simulink model "Dfig"  (R2017b)
settings: Solver=ode45  StartTime=0.0  StopTime=20  RelTol=1e-3  EnableMultiTasking=on
undefined symbols (not defined in the file): D, DiscIntNeverNeededParam, f, Fs, fsw, J, ki_id, ki_n, kp_id, kp_n, Lm, Lr, Ls, Lsi, p, Ps, Rr, Rs, sigma, Tem, Ts, Vbus, Vs
libraries: powerlib x8, powerlib_meascontrol x1
settings Model: Creator=admin  LastModifiedBy=admin
settings DataIOCC: LimitDataPoints=on  SaveFormat=Array
settings OptimizationCC: LifeSpan=inf
settings DebuggingCC: UnderspecifiedInitializationDetection=Classic  MergeDetectMultiDrivingBlocksExec=none  SolverPrmCheckMsg=warning  StateNameClashWarn=warning  SFUnexpectedBacktrackingDiag=warning  SFNoUnconditionalDefaultTransitionDiag=warning  SFExecutionAtInitializationDiag=none
settings HardwareCC: ProdBitPerPointer=32  ProdBitPerSizeT=32  ProdBitPerPtrDiffT=32  ProdLargestAtomicFloat=None  ProdIntDivRoundTo=Undefined  ProdEndianess=Unspecified  ProdWordSize=32  ProdHWDeviceType=32-bit Generic
settings ModelReferenceCC: PropagateSignalLabelsOutOfModel=off
settings CodeAppCC: StateflowObjectComments=on
settings GRTTargetCC: TargetLangStandard=C89/C90 (ANSI)  GeneratePreprocessorConditionals=Disable all
settings ConfigComp: CovMetricSettings=dw  CovHtmlReporting=on  CovSaveCumulativeToWorkspaceVar=on  CovSaveSingleToWorkspaceVar=on  CovExternalEMLEnable=off
settings SimscapeCC: SimscapeNormalizeSystem=off

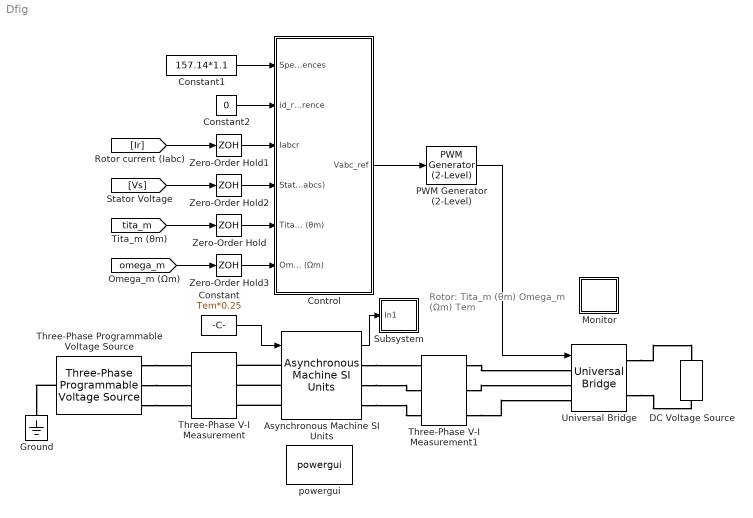
== system Dfig ==
  note: Rotor:
      | Tita_m (θm)
      | Omega_m (Ωm)
      | Tem
  Asynchronous Machine SI Units : powerlib/Machines/Asynchronous Machine SI Units  RotorType=Wound  PresetModel=No  MechanicalLoad=Torque Tm  ShowDetailedParameters=on  ReferenceFrame=Rotor  Units=SI  MeasurementBus=off  NominalParameters=[ Ps Vs f ]  Stator=[ Rs , Lsi]  Rotor=[ Rr , Lsi]  Cage1=[ 0.022 0.226/377]  Cage2=[ 0.022 0.226/377]  Lm=Lm  Mechanical=[ J D 2 ]  PolePairs=2  InitialConditions=[1 0 0 0 0 0 0 0]  SimulateSaturation=off  Saturation=[14.03593122, 27.81365428, 53.79336849, 72.68890987, 97.98006896, 148.6815601, 215.7428561, 302.9841135, 420.4778367 ; 230, 322, 414, 460, 506, 552, 598, 644, 690]  LoadFlowParameters=1492000  TsPowergui=0  TsBlock=-1  IterativeModel=Trapezoidal non iterative  IterativeDiscreteModel=Trapezoidal non iterative  Pmec=0
  Constant : Constant  Value=Tem*0.25
  Constant1 : Constant  Value=157.14*1.1
  Constant2 : Constant  Value=0
  Control : Subsystem
  DC Voltage Source : powerlib/Electrical Sources/DC Voltage Source  Amplitude=Vbus  Measurements=None
  Ground : powerlib/Elements/Ground  LConnTagsString=a
  Monitor : Subsystem
  PWM Generator (2-Level) : powerlib_meascontrol/Pulse & Signal Generators/PWM Generator (2-Level)  ModulatorType=Three-phase bridge (6 pulses)  ModulatorMode=Unsynchronized  Fc=fsw  Pc=90  nF=27  MinMax="[ -1  1 ]"  SamplingTechnique=Natural  ModulatingSignals=off  m=0.8  Freq=60  Phase=0  Ts=0  ShowCarrierOutport=off
      settings: SourceProductName=Simscape Power Systems
  Subsystem : Subsystem
  Three-Phase Programmable Voltage Source : powerlib/Electrical Sources/Three-Phase Programmable Voltage Source  PositiveSequence="[Vs  0 f]"  VariationEntity=None  VariationType=Table of time-amplitude pairs  VariationTypeAlt=Step  VariationStep=0.5  VariationRate=10  VariationMagnitude=0.3  VariationFrequency=2  VariationTiming=[1 2]  VariationPhaseA=off  Amplitudes=[1 0.8 1.2 1.0]  TimeValues=[0 0.1 0.15 0.2]  HarmonicGeneration=off  HarmonicA=[3 0.2 -25 0]  HarmonicB=[2 0.15 35 2]  Timing="[0.05  3]"  BusType=swing  Pref=0  Qref=0  Qmin=-inf  Qmax=inf
  Three-Phase V-I Measurement : powerlib/Measurements/Three-Phase V-I Measurement  VoltageMeasurement=phase-to-ground  SetLabelV=on  LabelV=Vs  Vpu=off  VpuLL=off  CurrentMeasurement=yes  SetLabelI=on  LabelI=Is  Ipu=off  Pbase=100e6  Vbase=500e3  OutputType=Complex  PhasorSimulation=off  PSBequivalent=0
  Three-Phase V-I Measurement1 : powerlib/Measurements/Three-Phase V-I Measurement  VoltageMeasurement=phase-to-phase  SetLabelV=on  LabelV=Vr  Vpu=off  VpuLL=off  CurrentMeasurement=yes  SetLabelI=on  LabelI=Ir  Ipu=off  Pbase=100e6  Vbase=500e3  OutputType=Complex  PhasorSimulation=off  PSBequivalent=0
  Universal Bridge : powerlib/Power Electronics/Universal Bridge  Arms=3  SnubberResistance=1e5  SnubberCapacitance=inf  Device=Ideal Switches  Ron=1e-3  Lon=0  ForwardVoltages="[  0  0  ]"  ForwardVoltage=0  GTOparameters=[ 10e-6 , 20e-6 ]  IGBTparameters=[ 1e-6 , 2e-6 ]  Measurements=None  Measurements_2=None  converterType=Rectifier
  Zero-Order Hold{,1..3} (4 alike) : ZeroOrderHold  SampleTime=1/fsw
  powergui : powerlib/powergui  Priority=1  SimulationMode=Discrete  SampleTime=Ts  frequency=60  Iterations=50  frequencyindice=50  Pbase=100e6  ErrMax=1e-4  UnitsV=kV  UnitsW=MW  buscounter=0  FunctionMessages=off  echomessages=off  EnableUseOfTLC=off  CurrentSourceSwitches=off  DisableSnubberDevices=off  DisableRonSwitches=off  DisableVfSwitches=off  DisplayEquations=off  SolverType=Tustin  Interpol=off  ExternalGateDelay=off  methode=off  Ts=0  x0status=blocks  SPID=off  SwTol=0  HookPort=off  RestoreLinks=warning  ResistiveCurrentMeasurement=off  Frange=[0:2:500]  Ylog=off  Xlog=on  ShowGrid=off  save=off  variable=ZData  structure=0  ZoomFFT=off  StartTime=0.0  cycles=1  DisplayStyle=1  fundamental=60  FreqAxis=off  MaxFrequency=1000  frequencyindicesteady=1  RmsSteady=1  display=off
  wires:
  Constant/1 -> Asynchronous Machine SI Units/1
  PWM Generator (2-Level)/1 -> Universal Bridge/1
  Control/1(Vabc_ref) -> PWM Generator (2-Level)/1
  Constant1/1 -> Control/1(Speed reference Omega_m (Ωm) references)
  Constant2/1 -> Control/2(id_reference)
  [Vs] -> Zero-Order Hold2/1
  [Ir] -> Zero-Order Hold1/1
  Asynchronous Machine SI Units/1 -> Subsystem/1(In1)
  [tita_m] -> Zero-Order Hold/1
  [omega_m] -> Zero-Order Hold3/1
  Zero-Order Hold1/1 -> Control/3(Iabcr)
  Zero-Order Hold2/1 -> Control/4(Stator Voltage (Vabcs))
  Zero-Order Hold/1 -> Control/5(Tita_m (θm))
  Zero-Order Hold3/1 -> Control/6(Omega_m (Ωm))
  connections:
  Three-Phase Programmable Voltage Source/LConn1 -- Ground/LConn1
  Three-Phase Programmable Voltage Source/RConn1 -- Three-Phase V-I Measurement/LConn1
  Three-Phase Programmable Voltage Source/RConn2 -- Three-Phase V-I Measurement/LConn2
  Three-Phase Programmable Voltage Source/RConn3 -- Three-Phase V-I Measurement/LConn3
  Asynchronous Machine SI Units/LConn1 -- Three-Phase V-I Measurement/RConn1
  Asynchronous Machine SI Units/LConn2 -- Three-Phase V-I Measurement/RConn2
  Asynchronous Machine SI Units/LConn3 -- Three-Phase V-I Measurement/RConn3
  Universal Bridge/RConn2 -- DC Voltage Source/LConn1
  Universal Bridge/RConn1 -- DC Voltage Source/RConn1
  Asynchronous Machine SI Units/RConn1 -- Three-Phase V-I Measurement1/RConn1
  Asynchronous Machine SI Units/RConn2 -- Three-Phase V-I Measurement1/RConn2
  Asynchronous Machine SI Units/RConn3 -- Three-Phase V-I Measurement1/RConn3
  Three-Phase V-I Measurement1/LConn1 -- Universal Bridge/LConn1
  Three-Phase V-I Measurement1/LConn2 -- Universal Bridge/LConn2
  Three-Phase V-I Measurement1/LConn3 -- Universal Bridge/LConn3

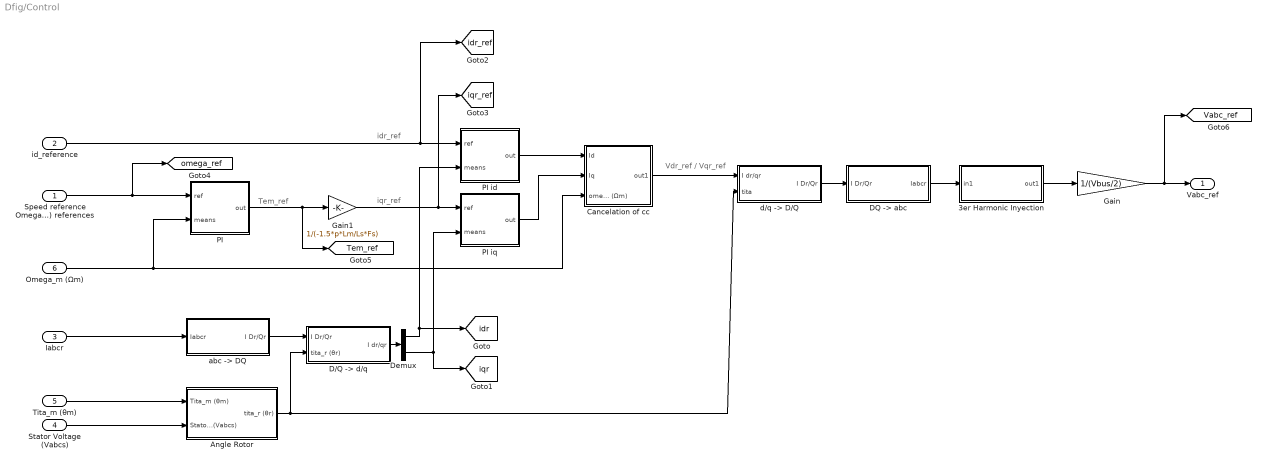
== system Dfig/Control ==
  note: Vdr_ref / Vqr_ref
  note: iqr_ref
  note: Tem_ref
  note: idr_ref
  Speed reference Omega_m (Ωm) references : Inport
  id_reference : Inport  Port=2
  Iabcr : Inport  Port=3
  Stator Voltage (Vabcs) : Inport  Port=4
  Tita_m (θm) : Inport  Port=5
  Omega_m (Ωm) : Inport  Port=6
  " Angle Rotor" : Subsystem
  3er Harmonic Inyection : Subsystem
  Cancelation of cc : Subsystem
  "D/Q -> d/q" : Subsystem
  "DQ -> abc" : Subsystem
  Demux : Demux  Outputs=2
  Gain : Gain  Gain=1/(Vbus/2)
  Gain1 : Gain  Gain=1/(-1.5*p*Lm/Ls*Fs)
  PI : Subsystem
  PI id : Subsystem
  PI iq : Subsystem
  "abc -> DQ " : Subsystem
  "d/q -> D/Q " : Subsystem
  Vabc_ref : Outport
  tag scope: Tem_ref=global, Vabc_ref=global, idr=global, idr_ref=global, iqr=global, iqr_ref=global, omega_ref=global
  wires:
  Gain/1 -> [Vabc_ref], Vabc_ref/1
  "DQ -> abc"/1(Iabcr) -> 3er Harmonic Inyection/1(in1)
  "d/q -> D/Q "/1(I Dr/Qr) -> "DQ -> abc"/1(I Dr/Qr)
  Iabcr/1 -> "abc -> DQ "/1(Iabcr)
  "abc -> DQ "/1(I Dr/Qr) -> "D/Q -> d/q"/1(I Dr/Qr)
  3er Harmonic Inyection/1(out1) -> Gain/1
  Tita_m (θm)/1 -> " Angle Rotor"/1(Tita_m (θm))
  Stator Voltage (Vabcs)/1 -> " Angle Rotor"/2(Stator Voltage (Vabcs))
  " Angle Rotor"/1(tita_r (θr)) -> "D/Q -> d/q"/2(tita_r (θr)), "d/q -> D/Q "/2(tita)
  PI id/1(out) -> Cancelation of cc/1(Id)
  PI iq/1(out) -> Cancelation of cc/2(Iq)
  Omega_m (Ωm)/1 -> PI/2(means), Cancelation of cc/3(omega_m (Ωm))
  "D/Q -> d/q"/1(I dr/qr) -> Demux/1
  Demux/2 -> [iqr], PI iq/2(means)
  Demux/1 -> [idr], PI id/2(means)
  Speed reference Omega_m (Ωm) references/1 -> PI/1(ref), [omega_ref]
  PI/1(out) -> [Tem_ref], Gain1/1
  Gain1/1 -> [iqr_ref], PI iq/1(ref)
  id_reference/1 -> [idr_ref], PI id/1(ref)
  Cancelation of cc/1(out1) -> "d/q -> D/Q "/1(I dr/qr)

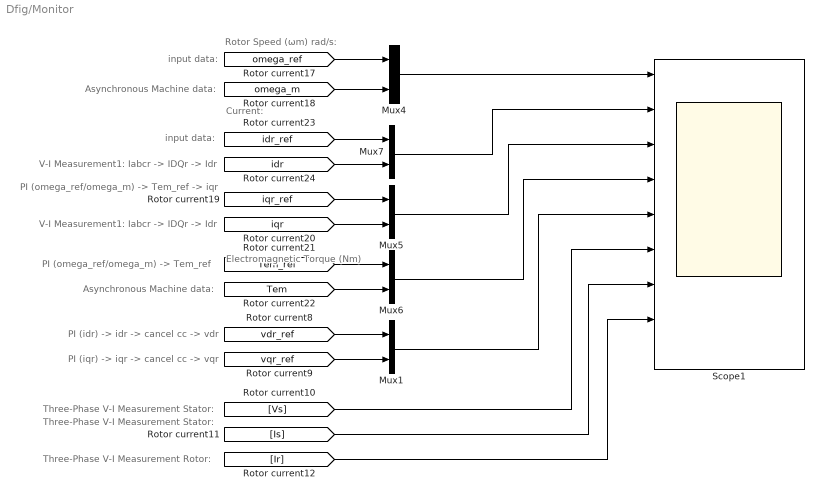
== system Dfig/Monitor ==
  note: Electromagnetic Torque (Nm)
  note: Three-Phase V-I Measurement Stator:
  note: PI (idr) -> idr -> cancel cc -> vdr
  note: PI (omega_ref/omega_m) -> Tem_ref -> iqr
  note: V-I Measurement1: Iabcr -> IDQr -> Idr
  note: input data:
  note: Current:
  note: Rotor Speed (ωm) rad/s:
  note: Asynchronous Machine data:
  note: input data:
  note: V-I Measurement1: Iabcr -> IDQr -> Idr
  note: PI (omega_ref/omega_m) -> Tem_ref
  note: Asynchronous Machine data:
  note: PI (iqr) -> iqr -> cancel cc -> vqr
  note: Three-Phase V-I Measurement Stator:
  note: Three-Phase V-I Measurement Rotor:
  Mux{1,4..7} (5 alike) : Mux  Inputs=2
  Scope1 : Scope  NumInputPorts=9
  wires:
  [omega_m] -> Mux4/2
  [omega_ref] -> Mux4/1
  [iqr_ref] -> Mux5/1
  [iqr] -> Mux5/2
  [Tem] -> Mux6/2
  [Tem_ref] -> Mux6/1
  [idr] -> Mux7/2
  [idr_ref] -> Mux7/1
  Mux4/1 -> Scope1/1
  [vdr_ref] -> Mux1/1
  [vqr_ref] -> Mux1/2
  Mux7/1 -> Scope1/2
  Mux5/1 -> Scope1/3
  Mux6/1 -> Scope1/4
  Mux1/1 -> Scope1/5
  [Vs] -> Scope1/6
  [Is] -> Scope1/7
  [Ir] -> Scope1/8

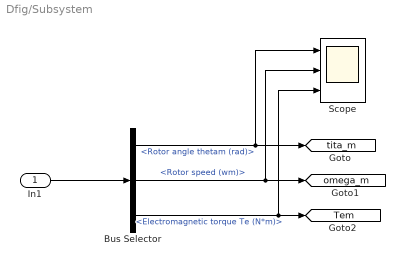
== system Dfig/Subsystem ==
  In1 : Inport
  Bus Selector : BusSelector  OutputSignals=Mechanical.Rotor angle thetam (rad),Mechanical.Rotor speed (wm),Mechanical.Electromagnetic torque Te (N*m)
  Scope : Scope  NumInputPorts=3
  tag scope: Tem=global, omega_m=global, tita_m=global
  wires:
  Bus Selector/2 -> Scope/2, [omega_m]  "<Rotor speed (wm)>"
  In1/1 -> Bus Selector/1
  Bus Selector/1 -> Scope/1, [tita_m]  "<Rotor angle thetam (rad)>"
  Bus Selector/3 -> Scope/3, [Tem]  "<Electromagnetic torque Te (N*m)>"

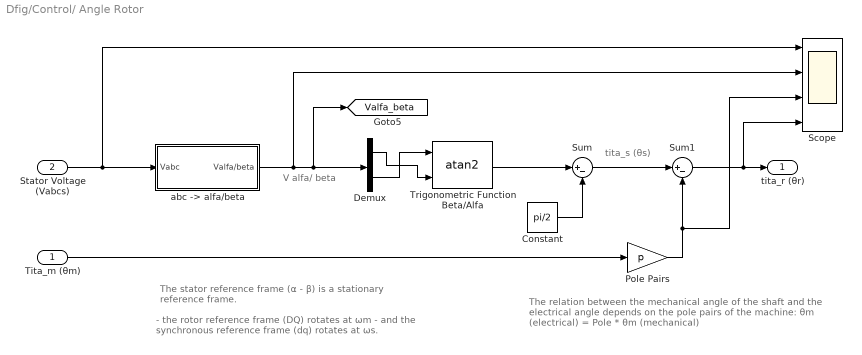
== system Dfig/Control/ Angle Rotor ==
  note: - the rotor reference frame (DQ) rotates at ωm
      | - and the synchronous reference frame (dq) rotates at ωs.
  note: The stator reference frame (α - β) is a stationary
      | reference frame.
  note: The relation between the mechanical angle of the shaft  and the
      | electrical angle depends on the pole pairs of the machine:
      |
      | θm (electrical) = Pole * θm (mechanical)
  note: tita_s (θs)
  note: V alfa/ beta
  Tita_m (θm) : Inport
  Stator Voltage (Vabcs) : Inport  Port=2
  Constant : Constant  Value=pi/2
  Demux : Demux  Outputs=2
  Pole Pairs : Gain  Gain=p
  Scope : Scope  NumInputPorts=4
  Sum : Sum  Inputs=|+-
  Sum1 : Sum  Inputs=|+-
  Trigonometric Function Beta/Alfa : Trigonometry  Operator=atan2
  "abc -> alfa/beta " : Subsystem
  tita_r (θr) : Outport
  tag scope: Valfa_beta=global
  wires:
  Stator Voltage (Vabcs)/1 -> Scope/1, "abc -> alfa/beta "/1(Vabc)
  Demux/2 -> Trigonometric Function Beta/Alfa/1
  Demux/1 -> Trigonometric Function Beta/Alfa/2
  "abc -> alfa/beta "/1("Valfa/beta ") -> Scope/2, [Valfa_beta], Demux/1
  Trigonometric Function Beta/Alfa/1 -> Sum/1
  Constant/1 -> Sum/2
  Tita_m (θm)/1 -> Pole Pairs/1
  Sum/1 -> Sum1/1
  Sum1/1 -> Scope/4, tita_r (θr)/1
  Pole Pairs/1 -> Sum1/2, Scope/3

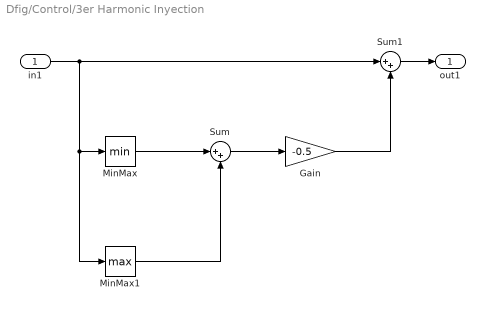
== system Dfig/Control/3er Harmonic Inyection ==
  in1 : Inport
  Gain : Gain  Gain=-0.5
  MinMax : MinMax
  MinMax1 : MinMax  Function=max
  Sum : Sum  Inputs=|++
  Sum1 : Sum  Inputs=|++
  out1 : Outport
  wires:
  in1/1 -> Sum1/1, MinMax1/1, MinMax/1
  MinMax/1 -> Sum/1
  MinMax1/1 -> Sum/2
  Sum1/1 -> out1/1
  Sum/1 -> Gain/1
  Gain/1 -> Sum1/2

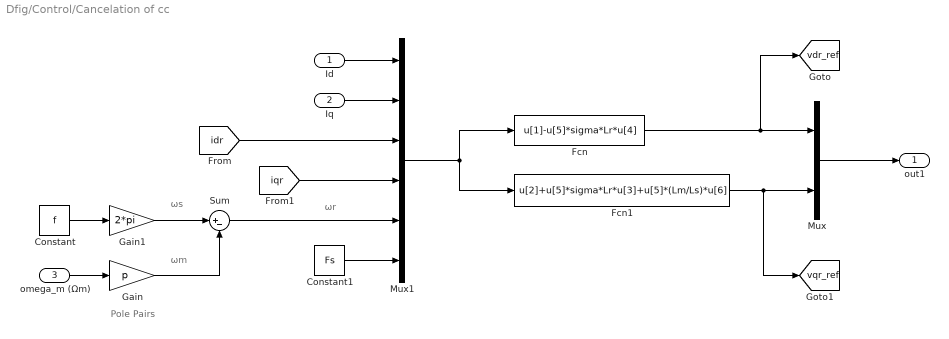
== system Dfig/Control/Cancelation of cc ==
  note: Pole Pairs
  note: ωr
  note: ωm
  note: ωs
  Id : Inport
  Iq : Inport  Port=2
  omega_m (Ωm) : Inport  Port=3
  Constant : Constant  Value=f
  Constant1 : Constant  Value=Fs
  Fcn : Fcn  Expr=u[1]-u[5]*sigma*Lr*u[4]
  Fcn1 : Fcn  Expr=u[2]+u[5]*sigma*Lr*u[3]+u[5]*(Lm/Ls)*u[6]
  Gain : Gain  Gain=p
  Gain1 : Gain  Gain=2*pi
  Mux : Mux  Inputs=2
  Mux1 : Mux  Inputs=6
  Sum : Sum  Inputs=|+-
  out1 : Outport
  tag scope: vdr_ref=global, vqr_ref=global
  wires:
  Mux/1 -> out1/1
  Fcn/1 -> [vdr_ref], Mux/1
  Fcn1/1 -> [vqr_ref], Mux/2
  Id/1 -> Mux1/1
  Iq/1 -> Mux1/2
  Mux1/1 -> Fcn1/1, Fcn/1
  [idr] -> Mux1/3
  [iqr] -> Mux1/4
  Constant1/1 -> Mux1/6
  omega_m (Ωm)/1 -> Gain/1
  Gain/1 -> Sum/2
  Constant/1 -> Gain1/1
  Gain1/1 -> Sum/1
  Sum/1 -> Mux1/5

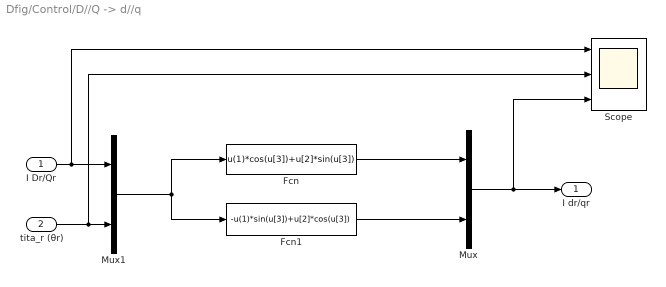
== system Dfig/Control/D//Q -> d//q ==
  I Dr/Qr : Inport
  tita_r (θr) : Inport  Port=2
  Fcn : Fcn  Expr=u(1)*cos(u[3])+u[2]*sin(u[3])
  Fcn1 : Fcn  Expr=-u(1)*sin(u[3])+u[2]*cos(u[3])
  Mux : Mux  Inputs=2
  Mux1 : Mux  Inputs=2
  Scope : Scope  NumInputPorts=3
  I dr/qr : Outport
  wires:
  Mux/1 -> Scope/3, I dr/qr/1
  Fcn/1 -> Mux/1
  Fcn1/1 -> Mux/2
  I Dr/Qr/1 -> Scope/1, Mux1/1
  tita_r (θr)/1 -> Scope/2, Mux1/2
  Mux1/1 -> Fcn/1, Fcn1/1

== system Dfig/Control/DQ -> abc ==
  I Dr/Qr : Inport
  Fcn : Fcn  Expr=u(1)
  Fcn1 : Fcn  Expr=-(u[1]/2)+u[2]*(sqrt(3)/2)
  Fcn2 : Fcn  Expr=-(u[1]/2)-u[2]*(sqrt(3)/2)
  Mux : Mux  Inputs=3
  Iabcr : Outport
  wires:
  Mux/1 -> Iabcr/1
  I Dr/Qr/1 -> Fcn2/1, Fcn1/1, Fcn/1
  Fcn/1 -> Mux/1
  Fcn1/1 -> Mux/2
  Fcn2/1 -> Mux/3

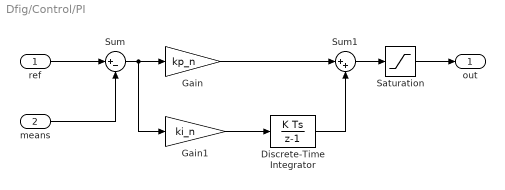
== system Dfig/Control/PI ==
  ref : Inport
  means : Inport  Port=2
  Discrete-Time Integrator : DiscreteIntegrator  SampleTime=1/fsw  LimitOutput=on  UpperSaturationLimit=Tem  LowerSaturationLimit=-Tem  ICPrevOutput=DiscIntNeverNeededParam  ICPrevScaledInput=DiscIntNeverNeededParam
  Gain : Gain  Gain=kp_n
  Gain1 : Gain  Gain=ki_n
  Saturation : Saturate  UpperLimit=Tem  LowerLimit=-Tem
  Sum : Sum  Inputs=|+-
  Sum1 : Sum  Inputs=|++
  out : Outport
  wires:
  means/1 -> Sum/2
  ref/1 -> Sum/1
  Sum/1 -> Gain1/1, Gain/1
  Gain/1 -> Sum1/1
  Gain1/1 -> Discrete-Time Integrator/1
  Discrete-Time Integrator/1 -> Sum1/2
  Sum1/1 -> Saturation/1
  Saturation/1 -> out/1

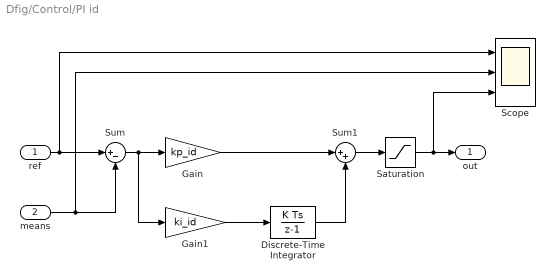
== system Dfig/Control/PI id ==
  ref : Inport
  means : Inport  Port=2
  Discrete-Time Integrator : DiscreteIntegrator  SampleTime=1/fsw  LimitOutput=on  UpperSaturationLimit=Vbus/sqrt(3)  LowerSaturationLimit=-Vbus/sqrt(3)  ICPrevOutput=DiscIntNeverNeededParam  ICPrevScaledInput=DiscIntNeverNeededParam
  Gain : Gain  Gain=kp_id
  Gain1 : Gain  Gain=ki_id
  Saturation : Saturate  UpperLimit=Vbus/sqrt(3)  LowerLimit=-Vbus/sqrt(3)
  Scope : Scope  NumInputPorts=3
  Sum : Sum  Inputs=|+-
  Sum1 : Sum  Inputs=|++
  out : Outport
  wires:
  means/1 -> Scope/2, Sum/2
  ref/1 -> Scope/1, Sum/1
  Sum/1 -> Gain1/1, Gain/1
  Gain/1 -> Sum1/1
  Gain1/1 -> Discrete-Time Integrator/1
  Discrete-Time Integrator/1 -> Sum1/2
  Sum1/1 -> Saturation/1
  Saturation/1 -> Scope/3, out/1

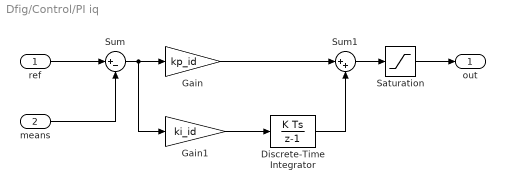
== system Dfig/Control/PI iq ==
  ref : Inport
  means : Inport  Port=2
  Discrete-Time Integrator : DiscreteIntegrator  SampleTime=1/fsw  LimitOutput=on  UpperSaturationLimit=Vbus/sqrt(3)  LowerSaturationLimit=-Vbus/sqrt(3)  ICPrevOutput=DiscIntNeverNeededParam  ICPrevScaledInput=DiscIntNeverNeededParam
  Gain : Gain  Gain=kp_id
  Gain1 : Gain  Gain=ki_id
  Saturation : Saturate  UpperLimit=Vbus/sqrt(3)  LowerLimit=-Vbus/sqrt(3)
  Sum : Sum  Inputs=|+-
  Sum1 : Sum  Inputs=|++
  out : Outport
  wires:
  means/1 -> Sum/2
  ref/1 -> Sum/1
  Sum/1 -> Gain1/1, Gain/1
  Gain/1 -> Sum1/1
  Gain1/1 -> Discrete-Time Integrator/1
  Discrete-Time Integrator/1 -> Sum1/2
  Sum1/1 -> Saturation/1
  Saturation/1 -> out/1

== system Dfig/Control/abc -> DQ  ==
  note: IQr
  note: IDr
  Iabcr : Inport
  Fcn : Fcn  Expr=2/3*(u[1]-u[2]/2-u[3]/2)
  Fcn1 : Fcn  Expr=2/3*(u[2]*(sqrt(3)/2)-u[3]*(sqrt(3)/2))
  Mux : Mux  Inputs=2
  Scope : Scope  NumInputPorts=2
  I Dr/Qr : Outport
  wires:
  Mux/1 -> Scope/2, I Dr/Qr/1
  Iabcr/1 -> Scope/1, Fcn1/1, Fcn/1
  Fcn/1 -> Mux/1
  Fcn1/1 -> Mux/2

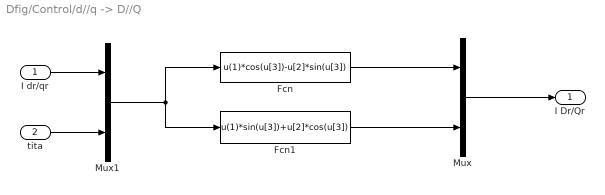
== system Dfig/Control/d//q -> D//Q  ==
  I dr/qr : Inport
  tita : Inport  Port=2
  Fcn : Fcn  Expr=u(1)*cos(u[3])-u[2]*sin(u[3])
  Fcn1 : Fcn  Expr=u(1)*sin(u[3])+u[2]*cos(u[3])
  Mux : Mux  Inputs=2
  Mux1 : Mux  Inputs=2
  I Dr/Qr : Outport
  wires:
  Mux/1 -> I Dr/Qr/1
  Fcn/1 -> Mux/1
  Fcn1/1 -> Mux/2
  I dr/qr/1 -> Mux1/1
  tita/1 -> Mux1/2
  Mux1/1 -> Fcn/1, Fcn1/1

== system Dfig/Control/ Angle Rotor/abc -> alfa//beta  ==
  Vabc : Inport
  Fcn : Fcn  Expr=2/3*(u[1]-u[2]/2-u[3]/2)
  Fcn1 : Fcn  Expr=2/3*(u[2]*(sqrt(3)/2)-u[3]*(sqrt(3)/2))
  Mux : Mux  Inputs=2
  "Valfa/beta " : Outport
  wires:
  Mux/1 -> "Valfa/beta "/1
  Vabc/1 -> Fcn1/1, Fcn/1
  Fcn/1 -> Mux/1
  Fcn1/1 -> Mux/2
